simulink model "SF049A_LoaMgr"  (R2013b)
settings: Solver=FixedStepDiscrete  SolverMode=SingleTasking  StartTime=0.0  StopTime=1  FixedStep=0.002  RelTol=1e-3
values from neighbouring files (symbols this model uses):
  CURRMEASLOAMTGTNMASK_CNT_U08 = DataDict.Constant    [SF049A_LoaMgr_DataDict.m]
  IVTRLOAMTGTNMASK_CNT_U08 = DataDict.Constant    [SF049A_LoaMgr_DataDict.m]
  LOAMAXSLEW_ULSPERSEC_F32 = DataDict.Constant    [SF049A_LoaMgr_DataDict.m]
  LoaMgrCurrIvtrMtgtnRate = DataDict.Calibration    [SF049A_LoaMgr_DataDict.m]
  LoaMgrCurrIvtrMtgtnSca = DataDict.Calibration    [SF049A_LoaMgr_DataDict.m]
  LoaMgrCurrIvtrMtgtnScaZeroEna = DataDict.Calibration    [SF049A_LoaMgr_DataDict.m]
  LoaMgrCurrMeasIdptSig0Resp = DataDict.Calibration    [SF049A_LoaMgr_DataDict.m]
  LoaMgrCurrMeasIdptSig1Resp = DataDict.Calibration    [SF049A_LoaMgr_DataDict.m]
  LoaMgrCurrMeasIdptSig2Resp = DataDict.Calibration    [SF049A_LoaMgr_DataDict.m]
  LoaMgrCurrMeasIdptSigFltThd = DataDict.Calibration    [SF049A_LoaMgr_DataDict.m]
  LoaMgrCurrMeasMtgtnRate = DataDict.Calibration    [SF049A_LoaMgr_DataDict.m]
  LoaMgrCurrMeasMtgtnSca = DataDict.Calibration    [SF049A_LoaMgr_DataDict.m]
  LoaMgrCurrMeasMtgtnScaZeroEna = DataDict.Calibration    [SF049A_LoaMgr_DataDict.m]
  LoaMgrFadeOutStRate = DataDict.Calibration    [SF049A_LoaMgr_DataDict.m]
  LoaMgrHwTqIdptSig0NoTqLoaResp = DataDict.Calibration    [SF049A_LoaMgr_DataDict.m]
  LoaMgrHwTqIdptSig1NoTqLoaResp = DataDict.Calibration    [SF049A_LoaMgr_DataDict.m]
  LoaMgrHwTqIdptSig2Resp = DataDict.Calibration    [SF049A_LoaMgr_DataDict.m]
  LoaMgrHwTqIdptSig4Resp = DataDict.Calibration    [SF049A_LoaMgr_DataDict.m]
  LoaMgrHwTqIdptSigFltThd = DataDict.Calibration    [SF049A_LoaMgr_DataDict.m]
  LoaMgrHwTqLoaAvlResp = DataDict.Calibration    [SF049A_LoaMgr_DataDict.m]
  LoaMgrIvtrIdptSig0Resp = DataDict.Calibration    [SF049A_LoaMgr_DataDict.m]
  LoaMgrIvtrIdptSig1Resp = DataDict.Calibration    [SF049A_LoaMgr_DataDict.m]
  LoaMgrIvtrIdptSig2Resp = DataDict.Calibration    [SF049A_LoaMgr_DataDict.m]
  LoaMgrIvtrIdptSigFltThd = DataDict.Calibration    [SF049A_LoaMgr_DataDict.m]
  LoaMgrIvtrMtgtnRate = DataDict.Calibration    [SF049A_LoaMgr_DataDict.m]
  LoaMgrIvtrMtgtnSca = DataDict.Calibration    [SF049A_LoaMgr_DataDict.m]
  LoaMgrIvtrMtgtnScaZeroEna = DataDict.Calibration    [SF049A_LoaMgr_DataDict.m]
  LoaMgrLimdStRate = DataDict.Calibration    [SF049A_LoaMgr_DataDict.m]
  LoaMgrLimdStSca = DataDict.Calibration    [SF049A_LoaMgr_DataDict.m]
  LoaMgrMotAgAvlSnsrlsResp = DataDict.Calibration    [SF049A_LoaMgr_DataDict.m]
  LoaMgrMotAgIdptSig0NoSnsrlsResp = DataDict.Calibration    [SF049A_LoaMgr_DataDict.m]
  LoaMgrMotAgIdptSig1NoSnsrlsResp = DataDict.Calibration    [SF049A_LoaMgr_DataDict.m]
  LoaMgrMotAgIdptSig2Resp = DataDict.Calibration    [SF049A_LoaMgr_DataDict.m]
  LoaMgrMotAgIdptSig3Resp = DataDict.Calibration    [SF049A_LoaMgr_DataDict.m]
  LoaMgrMotAgIdptSigFltThd = DataDict.Calibration    [SF049A_LoaMgr_DataDict.m]
  LoaMgrMotAgMtgtnRate = DataDict.Calibration    [SF049A_LoaMgr_DataDict.m]
  LoaMgrMotAgMtgtnSca = DataDict.Calibration    [SF049A_LoaMgr_DataDict.m]
  LoaMgrMotAgMtgtnScaZeroEna = DataDict.Calibration    [SF049A_LoaMgr_DataDict.m]
  LOASCAONE_ULS_F32 = DataDict.Constant    [SF049A_LoaMgr_DataDict.m]
  LOASCAZERO_ULS_F32 = DataDict.Constant    [SF049A_LoaMgr_DataDict.m]
  LOASTIMDTSHTDWN_CNT_U08 = DataDict.Constant    [SF049A_LoaMgr_DataDict.m]
  LOASTNORM_CNT_U08 = DataDict.Constant    [SF049A_LoaMgr_DataDict.m]
  LOASTSWMTGTN_CNT_U08 = DataDict.Constant    [SF049A_LoaMgr_DataDict.m]
  MAXCURRMEASIDPTSIGALLWD_CNT_U08 = DataDict.Constant    [SF049A_LoaMgr_DataDict.m]
  MAXHWTQIDPTSIGALLWD_CNT_U08 = DataDict.Constant    [SF049A_LoaMgr_DataDict.m]
  MAXIVTRIDPTSIGALLWD_CNT_U08 = DataDict.Constant    [SF049A_LoaMgr_DataDict.m]
  MAXMOTAGMECLIDPTSIGALLWD_CNT_U08 = DataDict.Constant    [SF049A_LoaMgr_DataDict.m]
  NODEBSTEP_CNT_U16 = DataDict.Constant    [SF049A_LoaMgr_DataDict.m]
undefined symbols (not defined in the file or in its folder): LoaSt1, NtcNr1, NtcSts1, SigQlfr1
libraries: simulink x43, NxtrMin x4, NxtrMax x4, NxtrLim x2
(part 8 of 8)

== system SF049A_LoaMgr/LoaMgr/LoaMgrPer1/Request_Responses/MotAgResp/one/cal1 ==
  In1 : Inport
  Action Port : ActionPort  ActionType=then
  CopyRight2 : Subsystem  Description=|  mask(Copyright Information){none=on}
      | Copyright info block.                                               
      |                                                                     
      | Place copyright information at the top of every subsystem in design.
      mask prompts: none "No parameters"
      mask help: Place copyright information at the top of every subsystem in design.
      mask Display:
      | NxtrConf = 'Nexteer Confidential';
      | 
      | sys = bdroot; %handle for the current model ("system")
      | first = get_param(sys,'Created');
      | first = first(end-3:end);  %year is last four digits
      | 
      | last = get_param(sys,'LastModifiedDate');
      | if isempty(last)
      |     last = datestr(now,'yyyy');
      | else
      |     last = last(end-3:end);
      | end
      | 
      | if strcmp(first,last)
      |     fprintf('%s -- Copyright %s Nexteer',NxtrConf,first)
      | else
      |     fprintf('%s -- %s%s- %s Nexteer',NxtrConf,char(169),first,last)
      | end
  Out2 : Outport
  wires:
  In1/1 -> Out2/1

== system SF049A_LoaMgr/LoaMgr/LoaMgrPer1/Request_Responses/MotAgResp/one/cal2 ==
  In1 : Inport
  Action Port : ActionPort  ActionType=else
  CopyRight2 : Subsystem  Description=|  mask(Copyright Information){none=on}
      | Copyright info block.                                               
      |                                                                     
      | Place copyright information at the top of every subsystem in design.
      mask prompts: none "No parameters"
      mask help: Place copyright information at the top of every subsystem in design.
      mask Display:
      | NxtrConf = 'Nexteer Confidential';
      | 
      | sys = bdroot; %handle for the current model ("system")
      | first = get_param(sys,'Created');
      | first = first(end-3:end);  %year is last four digits
      | 
      | last = get_param(sys,'LastModifiedDate');
      | if isempty(last)
      |     last = datestr(now,'yyyy');
      | else
      |     last = last(end-3:end);
      | end
      | 
      | if strcmp(first,last)
      |     fprintf('%s -- Copyright %s Nexteer',NxtrConf,first)
      | else
      |     fprintf('%s -- %s%s- %s Nexteer',NxtrConf,char(169),first,last)
      | end
  Out1 : Outport
  wires:
  In1/1 -> Out1/1

== system SF049A_LoaMgr/LoaMgr/LoaMgrPer1/Set_Faults/NTC_Fault1/SetNtcSts/CopyRight2 ==

== system SF049A_LoaMgr/LoaMgr/LoaMgrPer1/Set_Faults/NTC_Fault2/SetNtcSts/CopyRight2 ==

== system SF049A_LoaMgr/LoaMgr/LoaMgrPer1/Set_Faults/NTC_Fault3/SetNtcSts/CopyRight2 ==

== system SF049A_LoaMgr/LoaMgr/LoaMgrPer1/Set_Faults/NTC_Fault4/SetNtcSts/CopyRight2 ==

== system SF049A_LoaMgr/LoaMgr/LoaMgrPer1/Assign_Scale/SwMtgtn/OthersTrue/CurrIvtr/CopyRight2 ==

== system SF049A_LoaMgr/LoaMgr/LoaMgrPer1/Assign_Scale/SwMtgtn/OthersTrue/CurrIvtr/PassThru1 ==
  In1 : Inport
  In2 : Inport  Port=2
  Action Port : ActionPort  ActionType=then
  Sca : Outport
  Rate : Outport  Port=2
  wires:
  In1/1 -> Sca/1
  In2/1 -> Rate/1

== system SF049A_LoaMgr/LoaMgr/LoaMgrPer1/Assign_Scale/SwMtgtn/OthersTrue/CurrIvtr/PassThru2 ==
  In1 : Inport
  In2 : Inport  Port=2
  Action Port : ActionPort  ActionType=else
  Sca : Outport
  Rate : Outport  Port=2
  wires:
  In1/1 -> Sca/1
  In2/1 -> Rate/1

== system SF049A_LoaMgr/LoaMgr/LoaMgrPer1/Assign_Scale/SwMtgtn/OthersTrue/CurrOnly/CopyRight2 ==

== system SF049A_LoaMgr/LoaMgr/LoaMgrPer1/Assign_Scale/SwMtgtn/OthersTrue/CurrOnly/PassThru1 ==
  In1 : Inport
  In2 : Inport  Port=2
  Action Port : ActionPort  ActionType=then
  Sca : Outport
  Rate : Outport  Port=2
  wires:
  In1/1 -> Sca/1
  In2/1 -> Rate/1

== system SF049A_LoaMgr/LoaMgr/LoaMgrPer1/Assign_Scale/SwMtgtn/OthersTrue/CurrOnly/PassThru2 ==
  In1 : Inport
  In2 : Inport  Port=2
  Action Port : ActionPort  ActionType=else
  Sca : Outport
  Rate : Outport  Port=2
  wires:
  In1/1 -> Sca/1
  In2/1 -> Rate/1

== system SF049A_LoaMgr/LoaMgr/LoaMgrPer1/Assign_Scale/SwMtgtn/OthersTrue/Invalid_Number/CopyRight2 ==

== system SF049A_LoaMgr/LoaMgr/LoaMgrPer1/Assign_Scale/SwMtgtn/OthersTrue/IvtrOnly/CopyRight2 ==

== system SF049A_LoaMgr/LoaMgr/LoaMgrPer1/Assign_Scale/SwMtgtn/OthersTrue/IvtrOnly/PassThru1 ==
  In1 : Inport
  In2 : Inport  Port=2
  Action Port : ActionPort  ActionType=then
  Sca : Outport
  Rate : Outport  Port=2
  wires:
  In1/1 -> Sca/1
  In2/1 -> Rate/1

== system SF049A_LoaMgr/LoaMgr/LoaMgrPer1/Assign_Scale/SwMtgtn/OthersTrue/IvtrOnly/PassThru2 ==
  In1 : Inport
  In2 : Inport  Port=2
  Action Port : ActionPort  ActionType=else
  Sca : Outport
  Rate : Outport  Port=2
  wires:
  In1/1 -> Sca/1
  In2/1 -> Rate/1

== system SF049A_LoaMgr/LoaMgr/LoaMgrPer1/Request_Responses/HwTqResp/Zero_or_Invalid/cal1/CopyRight2 ==

== system SF049A_LoaMgr/LoaMgr/LoaMgrPer1/Request_Responses/HwTqResp/Zero_or_Invalid/cal2/CopyRight2 ==

== system SF049A_LoaMgr/LoaMgr/LoaMgrPer1/Request_Responses/HwTqResp/one/cal1/CopyRight2 ==

== system SF049A_LoaMgr/LoaMgr/LoaMgrPer1/Request_Responses/HwTqResp/one/cal2/CopyRight2 ==

== system SF049A_LoaMgr/LoaMgr/LoaMgrPer1/Request_Responses/MotAgResp/Zero_or_Invalid/cal1/CopyRight2 ==

== system SF049A_LoaMgr/LoaMgr/LoaMgrPer1/Request_Responses/MotAgResp/Zero_or_Invalid/cal2/CopyRight2 ==

== system SF049A_LoaMgr/LoaMgr/LoaMgrPer1/Request_Responses/MotAgResp/one/cal1/CopyRight2 ==

== system SF049A_LoaMgr/LoaMgr/LoaMgrPer1/Request_Responses/MotAgResp/one/cal2/CopyRight2 ==
